simulink model "VCMGCM1962020b_v2"  (R2020b)
settings: Solver=FixedStepDiscrete  StartTime=0.0  StopTime=10.0  FixedStep=0.005  RelTol=1e-3  EnableMultiTasking=on
PreLoadFcn:
  | try, model_open; catch, disp('Error occurred while executing model pre-load callback: model_open.m'); disp('Please assure that the MATLAB working directory is set to the model directory before opening.'); end
InitFcn:
  | try, model_open; catch, end
undefined symbols (not defined in the file): Bridge, GCM, H, raptor_get_param_eval, raptor_get_safe_string, raptor_xcp_function
libraries: Blocks_lib x1165, Raptor_lib x665, simulink x62, VCM_lib x5
(part 22 of 23)

== system VCMGCM1962020b_v2/Fgnd/Actuators/CAN/Battery/ChgrBatt_State_Transition_Cmd/MsgTx/doublestrike/Falling edge ==
  In : Inport
  AND6 : Logic  AllPortsSameDT=off  OutDataTypeStr=boolean
  NOT1 : Logic  Operator=NOT  AllPortsSameDT=off  OutDataTypeStr=boolean
  Unit Delay : UnitDelay  SampleTime=-1  HasFrameUpgradeWarning=on
  falling : Outport
  wires:
  AND6/1 -> falling/1
  In/1 -> Unit Delay/1, NOT1/1
  NOT1/1 -> AND6/1
  Unit Delay/1 -> AND6/2

== system VCMGCM1962020b_v2/Fgnd/Actuators/CAN/Battery/ChgrBatt_State_Transition_Cmd/MsgTx/doublestrike/rising edge ==
  In : Inport
  AND6 : Logic  AllPortsSameDT=off  OutDataTypeStr=boolean
  NOT1 : Logic  Operator=NOT  AllPortsSameDT=off  OutDataTypeStr=boolean
  Unit Delay : UnitDelay  SampleTime=-1  HasFrameUpgradeWarning=on
  rising : Outport
  wires:
  Unit Delay/1 -> AND6/1
  NOT1/1 -> AND6/2
  AND6/1 -> rising/1
  In/1 -> NOT1/1, Unit Delay/1

== system VCMGCM1962020b_v2/Fgnd/Actuators/CAN/Battery/ChgrBatt_State_Transition_Cmd/MsgTx/doublestrike/rising edge1 ==
  In : Inport
  AND6 : Logic  AllPortsSameDT=off  OutDataTypeStr=boolean
  NOT1 : Logic  Operator=NOT  AllPortsSameDT=off  OutDataTypeStr=boolean
  Unit Delay : UnitDelay  SampleTime=-1  HasFrameUpgradeWarning=on
  rising : Outport
  wires:
  Unit Delay/1 -> AND6/1
  NOT1/1 -> AND6/2
  AND6/1 -> rising/1
  In/1 -> NOT1/1, Unit Delay/1

== system VCMGCM1962020b_v2/Fgnd/Actuators/CAN/Other/A//C Compressor/MsgName/MsgTx/Key Start ==
  Data : Inport
  Bus Selector : BusSelector  OutputSignals=Control.Other.ACC.ACCEnblReq [Bool]
  Constant : Constant  Value=uint8(0)
  Constant1 : Constant  Value=uint8(3)
  Header : Blocks_lib/Header  width=Portrait  addtext=''
  Meas&Ovrd : Blocks_lib/Meas&Ovrd  nam=[nam 'KeyStart']  name_source=Parameter  view_as=Number  enum_struct={}  gain=1  min=-inf  max=inf  precision=''  units=''  help='CAN message value'  group=['Actuators | CAN | ' msgnam]
  Multiport Switch : MultiPortSwitch  DataPortOrder=Zero-based contiguous  Inputs=2  zeroidx=on  InputSameDT=on
  enum : Outport  VectorParamsAs1DForOutWhenUnconnected=off
  wires:
  Meas&Ovrd/1 -> enum/1
  Constant/1 -> Multiport Switch/2
  Multiport Switch/1 -> Meas&Ovrd/1
  Constant1/1 -> Multiport Switch/3
  Data/1 -> Bus Selector/1
  Bus Selector/1 -> Multiport Switch/1  "<ACCEnblReq [Bool]>"

== system VCMGCM1962020b_v2/Fgnd/Actuators/CAN/Other/Power Steering Pump Inverter/PSPInvtrHC1_Demands/MsgTx/Control Word ==
  Data : Inport
  3 == Energise : Constant  Value=uint8(3)
  5 == Enable : Constant  Value=uint8(5)
  6 == Shutdown : Constant  Value=uint8(6)
  7 == Energise : simulink/Logic and Bit Operations/Compare To Constant  relop===  const=7  OutDataTypeStr=boolean
  8 == Enable : simulink/Logic and Bit Operations/Compare To Constant  relop===  const=8  OutDataTypeStr=boolean
  Bus Selector : BusSelector  OutputSignals=Control.Other.PSPInvtr.PSPInvtrEnblReq [Bool],Sensors.CAN.Other.PSPInvtr.PSPInvtrHS2_Status_Feedback.PSPInvtrInverterStatus.PSPInvtrInverterStatus [enum]
  Header : Blocks_lib/Header  width=Portrait  addtext=''
  Logical Operator : Logic  Operator=OR  OutDataTypeStr=boolean
  Meas&Ovrd : Blocks_lib/Meas&Ovrd  nam=[nam 'ControlWord']  name_source=Parameter  view_as=Number  enum_struct={}  gain=1  min=-inf  max=inf  precision=''  units='-'  help='CAN message value'  group=['Actuators | CAN | ' msgnam]
  Multiport Switch : MultiPortSwitch  DataPortOrder=Zero-based contiguous  Inputs=2  zeroidx=on  InputSameDT=on
  Multiport Switch1 : MultiPortSwitch  DataPortOrder=Zero-based contiguous  Inputs=2  zeroidx=on  InputSameDT=on
  enum : Outport  VectorParamsAs1DForOutWhenUnconnected=off
  wires:
  6 == Shutdown/1 -> Multiport Switch1/2
  Bus Selector/1 -> Multiport Switch1/1  "<PSPInvtrEnblReq [Bool]>"
  Multiport Switch/1 -> Multiport Switch1/3
  Multiport Switch1/1 -> Meas&Ovrd/1
  Logical Operator/1 -> Multiport Switch/1
  8 == Enable/1 -> Logical Operator/2
  3 == Energise/1 -> Multiport Switch/2
  5 == Enable/1 -> Multiport Switch/3
  7 == Energise/1 -> Logical Operator/1
  Bus Selector/2 -> 8 == Enable/1, 7 == Energise/1  "<PSPInvtrInverterStatus [enum]>"
  Meas&Ovrd/1 -> enum/1
  Data/1 -> Bus Selector/1

== system VCMGCM1962020b_v2/Fgnd/Control/Drive Inverter/Motor Torque Request/Driver Torque Request/Cruise Control/Control/Arbitration State ==
  PedTrq : Inport
  PIReq : Inport  Port=2
  Add : Sum
  Header : Blocks_lib/Header  width=Portrait  addtext=''
  Mux : Mux  Inputs=2
  RelOp(w/Hyst) : Blocks_lib/RelOp(w//Hyst)  relop=>=
  raptor_adjustment1 : Raptor_lib/Data Storage/raptor_adjustment  paramName='CCPedalArbHyst'  nameSource=Parameter  initValue=0  dataType=double  storage=Calibration  calDispType=Number  calEnum={}  calGain=1  calOffset=0  calMax=inf  calMin=-inf  calFormat=''  calUnit='Nm'  calHelp='Hysteresis used to determine arbitration'  calAccess=1  calFunction=group  calDispHeaders=off  calColHeaders={'Col1' 'Col2' 'Col3'}  calRowHeaders={'Row1' 'Row2' 'Row3'}
      settings: SourceProductName=Raptor
  raptor_measurement1 : Raptor_lib/Data Storage/raptor_measurement  paramName='CCPedalWinArb'  nameSource=Parameter  calDispType=Number  calEnum={'Not adapting', 'Adapting'}  calGain=1  calOffset=0  calMax=inf  calMin=-inf  calFormat=''  calUnit='Bool'  calHelp='Pedal winning arbitraion (while in cruise control)'  calAccess=1  calFunction=group  calVisible=on
      settings: SourceProductName=Raptor
  "PedWinArb " : Outport  VectorParamsAs1DForOutWhenUnconnected=off
  wires:
  RelOp(w/Hyst)/1 -> "PedWinArb "/1, raptor_measurement1/1
  PIReq/1 -> Add/2, Mux/2
  PedTrq/1 -> RelOp(w/Hyst)/1
  raptor_adjustment1/1 -> Add/1
  Add/1 -> Mux/1
  Mux/1 -> RelOp(w/Hyst)/2

== system VCMGCM1962020b_v2/Fgnd/Control/Drive Inverter/Motor Torque Request/Driver Torque Request/Cruise Control/Control/PICtrl(w//VarGain)(w//ICInport)(w//AntiWindup) ==
  Setpt : Inport
  Act : Inport  Port=2
  Rst : Inport  Port=3
  IC : Inport  Port=4
  Hold : Inport  Port=5
  Mx : Inport  Port=6
  Mn : Inport  Port=7
  Header : Blocks_lib/Header  width=Portrait  addtext=''
  PI(w/AntiWindup)(w/Hold) : Subsystem  mask(PI){samptime=samptime}
      mask prompts: samptime "Sample Time (sec)"
      mask Display: disp('PI');
  raptor_calibration1 : Raptor_lib/Data Storage/raptor_adjustment  paramName=[nam 'ErrGain']  nameSource=Parameter  initValue=0  dataType=double  storage=Calibration  calDispType=Number  calEnum={'Disabled', 'Enabled'}  calGain=1  calOffset=0  calMax=inf  calMin=-inf  calFormat=''  calUnit=[units '/' inunits]  calHelp='PID controller error gain'  calAccess=1  calFunction=group  calDispHeaders=off  calColHeaders={'Col1' 'Col2' 'Col3'}  calRowHeaders={'Row1' 'Row2' 'Row3'}
      settings: SourceProductName=Raptor
  raptor_data_def : Raptor_lib/Data Storage/raptor_data_def  dataName=[nam 'ITrm']  initValue=0  dataType=double  storage=Volatile (RAM)  calVisible=on  calType=Measurement  calDispType=Number  calEnum={'Disabled', 'Enabled'}  calGain=1  calOffset=0  calMin=-inf  calMax=inf  calFormat=''  calUnit=units  calHelp='PID controller integral term'  calAccess=1  calFunction=group  calDispHeaders=off  calColHeaders={'Col1' 'Col2' 'Col3'}  calRowHeaders={'Row1' 'Row2' 'Row3'}
      settings: SourceProductName=Raptor
  raptor_data_read : Raptor_lib/Data Storage/raptor_data_read  dataName=[nam 'ITrm']  dataShape=Scalar  idxSource=Input  idxRow=1  idxCol=1
      settings: SourceProductName=Raptor
  raptor_data_write : Raptor_lib/Data Storage/raptor_data_write  dataName=[nam 'ITrm']  dataShape=Scalar  idxSource=Write Entire Vector/Matrix  idxRow=1  idxCol=1
      settings: SourceProductName=Raptor
  raptor_interpolation_1d : Raptor_lib/Table Lookup/raptor_table_interpolate_1d  dataName=[nam 'PGainTbl']  initValue=zeros(1,dim(1))  dataType=double  storage=Calibration  adapt=off  adaptMode=Adapt between points  adaptOut=off  calVisible=on  calGain=1  calOffset=0  calMax=inf  calMin=-inf  calFormat='0.3'  calUnit='-'  calHelp='PID controller proportional gain'  calAccess=1  calFunction=group  measureEnable=on  mName=[nam 'PGain']
      settings: SourceProductName=Raptor
  raptor_interpolation_1d1 : Raptor_lib/Table Lookup/raptor_table_interpolate_1d  dataName=[nam 'IGainTbl']  initValue=zeros(1,dim(1))  dataType=double  storage=Calibration  adapt=off  adaptMode=Adapt between points  adaptOut=off  calVisible=on  calGain=1  calOffset=0  calMax=inf  calMin=-inf  calFormat='0.3'  calUnit='1/sec'  calHelp='PID controller integral gain'  calAccess=1  calFunction=group  measureEnable=on  mName=[nam 'IGain']
      settings: SourceProductName=Raptor
  raptor_prelookup4 : Raptor_lib/Table Lookup/raptor_table_axis  dataName=[nam 'Err' num2str(dim(1)) 'IdxArr']  initValue=[1:dim(1)]  dataType=double  storage=Calibration  calVisible=on  calGain=1  calOffset=0  calMax=inf  calMin=-inf  calFormat=''  calUnit=inunits  calHelp='Index array'  calAccess=1  calFunction=group
      settings: SourceProductName=Raptor
  raptor_probe : Raptor_lib/Data Storage/raptor_measurement  paramName=[nam 'ErrTrm']  nameSource=Parameter  calDispType=Number  calEnum={'Disabled', 'Enabled'}  calGain=1  calOffset=0  calMax=inf  calMin=-inf  calFormat=''  calUnit=inunits  calHelp='PID controller error term'  calAccess=1  calFunction=group  calVisible=on
      settings: SourceProductName=Raptor
  raptor_probe1 : Raptor_lib/Data Storage/raptor_measurement  paramName=[nam 'PTrm']  nameSource=Parameter  calDispType=Number  calEnum={'Disabled', 'Enabled'}  calGain=1  calOffset=0  calMax=inf  calMin=-inf  calFormat=''  calUnit=units  calHelp='PID controller proportional term'  calAccess=1  calFunction=group  calVisible=on
      settings: SourceProductName=Raptor
  raptor_probe6 : Raptor_lib/Data Storage/raptor_measurement  paramName=[nam 'Cmd']  nameSource=Parameter  calDispType=Number  calEnum={'Disabled', 'Enabled'}  calGain=1  calOffset=0  calMax=inf  calMin=-inf  calFormat=''  calUnit=units  calHelp='PID controller output'  calAccess=1  calFunction=group  calVisible=on
      settings: SourceProductName=Raptor
  Cmd : Outport  VectorParamsAs1DForOutWhenUnconnected=off
  wires:
  Rst/1 -> PI(w/AntiWindup)(w/Hold)/6(Rst)
  Act/1 -> PI(w/AntiWindup)(w/Hold)/2(Act)
  Setpt/1 -> PI(w/AntiWindup)(w/Hold)/1(Setpt)
  raptor_calibration1/1 -> PI(w/AntiWindup)(w/Hold)/3(kErr)
  IC/1 -> PI(w/AntiWindup)(w/Hold)/7(IC)
  PI(w/AntiWindup)(w/Hold)/3(PTerm) -> raptor_probe1/1
  PI(w/AntiWindup)(w/Hold)/1(Out) -> Cmd/1, raptor_probe6/1
  raptor_interpolation_1d/1 -> PI(w/AntiWindup)(w/Hold)/4(kP)
  raptor_interpolation_1d1/1 -> PI(w/AntiWindup)(w/Hold)/5(kI)
  raptor_prelookup4/1 -> raptor_interpolation_1d/1, raptor_interpolation_1d1/1
  raptor_data_read/1 -> PI(w/AntiWindup)(w/Hold)/11(PrevITrm)
  PI(w/AntiWindup)(w/Hold)/4(ITrm) -> raptor_data_write/1
  PI(w/AntiWindup)(w/Hold)/2(Err) -> raptor_prelookup4/1, raptor_probe/1
  Mx/1 -> PI(w/AntiWindup)(w/Hold)/9(Mx)
  Mn/1 -> PI(w/AntiWindup)(w/Hold)/10(Mn)
  Hold/1 -> PI(w/AntiWindup)(w/Hold)/8(Hold)

== system VCMGCM1962020b_v2/Fgnd/Control/Drive Inverter/Motor Torque Request/Driver Torque Request/Cruise Control/Control/Reset, IC, & Limits ==
  note: Note: This is the previous time-step
      | final torque request.
  note: Note:
      | On the first time step (ie, cruise control becoming active), the integral term is pre-loaded at (LastTrqReq - FFTerm).
      | Then, when the feedforward term and PTerm is added, the initial output of the complete controller is (LastTrqReq + PTerm).
      |
      | When the pedal is winning arbitration , the idle PI controller’s integral term is also reset to (LastTrqReq – FFTerm).
      | Then, when the feedforward term and PTerm is added, the output of the complete controller is (LastTrqReq + PTerm).
  Data : Inport
  Setpt : Inport  Port=2
  FF : Inport  Port=3
  PedWinArb : Inport  Port=4
  Add1 : Sum  Inputs=+-
  Add2 : Sum  Inputs=+-
  Add3 : Sum  Inputs=+-
  Bus Selector : BusSelector  OutputSignals=Control.DrvInvtr.MtrTrqReq.DrvInvtr.DrvMtrTrqLim [Nm]
  Bus Selector1 : BusSelector  OutputSignals=Control.DrvInvtr.MtrTrqReq.DrvInvtr.DrvMtrTrqReq [Nm]
  Demux : Demux  Outputs=2
  FirstTS : Blocks_lib/FirstTS  SystemSampleTime=-1  VariantActivationTime=update diagram  Latency=0  AutoFrameSizeCalculation=off
  Header : Blocks_lib/Header  width=Portrait  addtext=''
  Logical Operator : Logic  Operator=OR  AllPortsSameDT=off  OutDataTypeStr=boolean
  Speed Pulled High : Subsystem
  Unit Delay : UnitDelay  SampleTime=-1  HasFrameUpgradeWarning=on
  Rst : Outport  VectorParamsAs1DForOutWhenUnconnected=off
  " IC " : Outport  Port=2  VectorParamsAs1DForOutWhenUnconnected=off
  " Hold" : Outport  Port=3  VectorParamsAs1DForOutWhenUnconnected=off
  Mx : Outport  Port=4  VectorParamsAs1DForOutWhenUnconnected=off
  Mn : Outport  Port=5  VectorParamsAs1DForOutWhenUnconnected=off
  wires:
  Unit Delay/1 -> Add1/1
  Add3/1 -> Mn/1
  Bus Selector1/1 -> Unit Delay/1  "<DrvMtrTrqReq [Nm]>"
  Add2/1 -> Mx/1
  Add1/1 -> " IC "/1
  Demux/1 -> Add2/1
  FirstTS/1 -> Logical Operator/1
  FF/1 -> Add1/2, Add3/2, Add2/2
  PedWinArb/1 -> Logical Operator/2, Speed Pulled High/3(PedWinArb)
  Logical Operator/1 -> Rst/1
  Speed Pulled High/1(Bool) -> " Hold"/1
  Setpt/1 -> Speed Pulled High/2(Setpt)
  Demux/2 -> Add3/1
  Bus Selector/1 -> Demux/1  "<DrvMtrTrqLim [Nm]>"
  Data/1 -> Bus Selector1/1, Speed Pulled High/1(Data), Bus Selector/1

== system VCMGCM1962020b_v2/Fgnd/Control/Drive Inverter/Motor Torque Request/Driver Torque Request/Cruise Control/Setpoint/Enable ==
  Data : Inport
  Bus Selector : BusSelector  OutputSignals=Control.Mode.PRNDMode [enum]
  Bus Selector1 : BusSelector  OutputSignals=VirtualSensors.Spd.VehDir [enum]
  Bus Selector2 : BusSelector  OutputSignals=VirtualSensors.Spd.VehSpd [kph]
  CmprTo : Blocks_lib/CmprTo  op===  val='Drv'  enum=EnumLst.PRNDMode
  CmprTo1 : Blocks_lib/CmprTo  op===  val='Fwd'  enum=EnumLst.VehDir
  Header : Blocks_lib/Header  width=Portrait  addtext=''
  Logical Operator : Logic  Inputs=1  OutDataTypeStr=boolean
  Logical Operator1 : Logic  Operator=NOT  Inputs=1  OutDataTypeStr=boolean
  Mux : Mux  Inputs=5
  Relational Operator : RelationalOperator  Operator=<=  OutDataTypeStr=boolean  RndMeth=Simplest
  raptor_adjustment : Raptor_lib/Data Storage/raptor_adjustment  paramName='CCEnbl_cal'  nameSource=Parameter  initValue=0  dataType=boolean  storage=Calibration  calDispType=Number  calEnum={'False', 'True'}  calGain=1  calOffset=0  calMax=inf  calMin=-inf  calFormat=''  calUnit='Bool'  calHelp='Cruise control enable'  calAccess=1  calFunction=group  calDispHeaders=off  calColHeaders={'Col1' 'Col2' 'Col3'}  calRowHeaders={'Row1' 'Row2' 'Row3'}
      settings: SourceProductName=Raptor
  raptor_adjustment1 : Raptor_lib/Data Storage/raptor_adjustment  paramName='CCVehSpdHiThr'  nameSource=Parameter  initValue=0  dataType=double  storage=Calibration  calDispType=Number  calEnum={'False', 'True'}  calGain=1  calOffset=0  calMax=inf  calMin=-inf  calFormat=''  calUnit='kph'  calHelp='Cruise control enable vehicle speed high threshold'  calAccess=1  calFunction=group  calDispHeaders=off  calColHeaders={'Col1' 'Col2' 'Col3'}  calRowHeaders={'Row1' 'Row2' 'Row3'}
      settings: SourceProductName=Raptor
  raptor_fault_action : Raptor_lib/Faults/raptor_fault_action  actionName='CCDsbl'  calVisible=off  calAccess=1  calFunction='System | FaultManager | FaultAction'
      settings: SourceProductName=Raptor
  raptor_measurement : Raptor_lib/Data Storage/raptor_measurement  paramName='CCEnbl'  nameSource=Parameter  calDispType=Number  calEnum={}  calGain=1  calOffset=0  calMax=inf  calMin=-inf  calFormat=''  calUnit='Bool'  calHelp='Cruise control enable criteria met'  calAccess=1  calFunction=group  calVisible=on
      settings: SourceProductName=Raptor
  Enbl : Outport  VectorParamsAs1DForOutWhenUnconnected=off
  wires:
  CmprTo/1 -> Mux/3
  Bus Selector/1 -> CmprTo/1  "<PRNDMode [enum]>"
  Mux/1 -> raptor_measurement/1, Logical Operator/1
  Relational Operator/1 -> Mux/5
  raptor_adjustment1/1 -> Relational Operator/2
  raptor_adjustment/1 -> Mux/1
  Bus Selector2/1 -> Relational Operator/1  "<VehSpd [kph]>"
  Logical Operator1/1 -> Mux/2
  Logical Operator/1 -> Enbl/1
  raptor_fault_action/1 -> Logical Operator1/1
  Data/1 -> Bus Selector/1, Bus Selector1/1, Bus Selector2/1
  Bus Selector1/1 -> CmprTo1/1  "<VehDir [enum]>"
  CmprTo1/1 -> Mux/4

== system VCMGCM1962020b_v2/Fgnd/Control/Drive Inverter/Motor Torque Request/Driver Torque Request/Cruise Control/Setpoint/SetptMnMx ==
  Data : Inport
  Add : Sum  Inputs=+-
  Add1 : Sum
  Bus Selector : BusSelector  OutputSignals=Control.DrvInvtr.MtrTrqReq.DrvTrqReq.VehSpdLim [kph]
  Header : Blocks_lib/Header  width=Portrait  addtext=''
  MinMax : MinMax  Inputs=2
  raptor_adjustment : Raptor_lib/Data Storage/raptor_adjustment  paramName='CCSetptMnMxDelta'  nameSource=Parameter  initValue=0  dataType=double  storage=Calibration  calDispType=Number  calEnum={'False', 'True'}  calGain=1  calOffset=0  calMax=inf  calMin=-inf  calFormat=''  calUnit='kph'  calHelp='Cruise control setpoint minimum/maximum delta (relative to high/low thresholds)'  calAccess=1  calFunction=group  calDispHeaders=off  calColHeaders={'Col1' 'Col2' 'Col3'}  calRowHeaders={'Row1' 'Row2' 'Row3'}
      settings: SourceProductName=Raptor
  raptor_data_read : Raptor_lib/Data Storage/raptor_data_read  dataName='CCVehSpdLoThr'  dataShape=Scalar  idxSource=Read Entire Vector/Matrix  idxRow=1  idxCol=1
      settings: SourceProductName=Raptor
  raptor_data_read1 : Raptor_lib/Data Storage/raptor_data_read  dataName='CCVehSpdHiThr'  dataShape=Scalar  idxSource=Read Entire Vector/Matrix  idxRow=1  idxCol=1
      settings: SourceProductName=Raptor
  Mx : Outport  VectorParamsAs1DForOutWhenUnconnected=off
  Mn : Outport  Port=2  VectorParamsAs1DForOutWhenUnconnected=off
  wires:
  raptor_adjustment/1 -> Add/2, Add1/1
  Add/1 -> MinMax/2
  Bus Selector/1 -> MinMax/1  "<VehSpdLim [kph]>"
  Data/1 -> Bus Selector/1
  Add1/1 -> Mn/1
  MinMax/1 -> Mx/1
  raptor_data_read/1 -> Add1/2
  raptor_data_read1/1 -> Add/1

== system VCMGCM1962020b_v2/Fgnd/Control/Drive Inverter/Motor Torque Request/Driver Torque Request/Cruise Control/Setpoint/Standby ==
  Data : Inport
  Bus Selector : BusSelector  OutputSignals=VirtualSensors.Driver.BrkSw [Bool]
  Bus Selector1 : BusSelector  OutputSignals=VirtualSensors.Driver.CCCancel [Bool]
  Bus Selector2 : BusSelector  OutputSignals=VirtualSensors.Spd.VehSpd [kph]
  Header : Blocks_lib/Header  width=Portrait  addtext=''
  Logical Operator : Logic  Operator=OR  Inputs=1  OutDataTypeStr=boolean
  Mux : Mux  Inputs=3
  Relational Operator : RelationalOperator  Operator=<  OutDataTypeStr=boolean  RndMeth=Simplest
  raptor_adjustment : Raptor_lib/Data Storage/raptor_adjustment  paramName='CCVehSpdLoThr'  nameSource=Parameter  initValue=0  dataType=double  storage=Calibration  calDispType=Number  calEnum={'False', 'True'}  calGain=1  calOffset=0  calMax=inf  calMin=-inf  calFormat=''  calUnit='kph'  calHelp='Cruise control enable vehicle speed low threshold'  calAccess=1  calFunction=group  calDispHeaders=off  calColHeaders={'Col1' 'Col2' 'Col3'}  calRowHeaders={'Row1' 'Row2' 'Row3'}
      settings: SourceProductName=Raptor
  raptor_measurement : Raptor_lib/Data Storage/raptor_measurement  paramName='CCStndby'  nameSource=Parameter  calDispType=Number  calEnum={}  calGain=1  calOffset=0  calMax=inf  calMin=-inf  calFormat=''  calUnit='Bool'  calHelp='Cruise control in standby'  calAccess=1  calFunction=group  calVisible=on
      settings: SourceProductName=Raptor
  Stndby : Outport  VectorParamsAs1DForOutWhenUnconnected=off
  wires:
  Bus Selector1/1 -> Mux/2  "<CCCancel [Bool]>"
  Logical Operator/1 -> Stndby/1
  raptor_adjustment/1 -> Relational Operator/2
  Bus Selector2/1 -> Relational Operator/1  "<VehSpd [kph]>"
  Bus Selector/1 -> Mux/1  "<BrkSw [Bool]>"
  Relational Operator/1 -> Mux/3
  Mux/1 -> raptor_measurement/1, Logical Operator/1
  Data/1 -> Bus Selector/1, Bus Selector1/1, Bus Selector2/1

== system VCMGCM1962020b_v2/Fgnd/Control/Drive Inverter/Motor Torque Request/Inverter//Motor Limit & Request/Motor Torque Request/Gearbox Preload/Preload Initialize ==
  Data : Inport
  TrqReq : Inport  Port=2
  Bus Selector : BusSelector  OutputSignals=Control.Mode.PRNDMode [enum]
  CmprTo : Blocks_lib/CmprTo  op===  val='Rev'  enum=EnumLst.PRNDMode
  CmprTo1 : Blocks_lib/CmprTo  op===  val='Drv'  enum=EnumLst.PRNDMode
  Combinatorial Logic : CombinatorialLogic  TruthTable=[0; 2; 1; 0]
  Compare To Zero : simulink/Logic and Bit Operations/Compare To Zero  relop=<=  OutDataTypeStr=boolean
  Compare To Zero1 : simulink/Logic and Bit Operations/Compare To Zero  relop=>=  OutDataTypeStr=boolean
  Detect Increase{,1..3} (4 alike) : simulink/Logic and Bit Operations/Detect Increase  vinit=0.0  OutDataTypeStr=boolean
  Header : Blocks_lib/Header  width=Portrait  addtext=''
  Logical Operator : Logic  Operator=OR  AllPortsSameDT=off  OutDataTypeStr=boolean
  Logical Operator1 : Logic  AllPortsSameDT=off  OutDataTypeStr=boolean
  Logical Operator2 : Logic  Operator=OR  AllPortsSameDT=off  OutDataTypeStr=boolean
  Logical Operator3 : Logic  AllPortsSameDT=off  OutDataTypeStr=boolean
  Mux : Mux  Inputs=2
  enum : Outport  VectorParamsAs1DForOutWhenUnconnected=off
  wires:
  CmprTo1/1 -> Logical Operator3/1, Detect Increase1/1
  CmprTo/1 -> Logical Operator1/1, Detect Increase/1
  Logical Operator/1 -> Mux/1
  Logical Operator2/1 -> Mux/2
  Logical Operator3/1 -> Logical Operator2/2
  Compare To Zero1/1 -> Detect Increase3/1
  Detect Increase3/1 -> Logical Operator3/2
  Detect Increase2/1 -> Logical Operator1/2
  Compare To Zero/1 -> Detect Increase2/1
  TrqReq/1 -> Compare To Zero/1, Compare To Zero1/1
  Logical Operator1/1 -> Logical Operator/2
  Combinatorial Logic/1 -> enum/1
  Mux/1 -> Combinatorial Logic/1
  Detect Increase1/1 -> Logical Operator2/1
  Detect Increase/1 -> Logical Operator/1
  Data/1 -> Bus Selector/1
  Bus Selector/1 -> CmprTo1/1, CmprTo/1  "<PRNDMode [enum]>"

== system VCMGCM1962020b_v2/Fgnd/Control/Drive Inverter/Motor Torque Request/Inverter//Motor Limit & Request/Motor Torque Request/Rate Limit/RateLim ==
  Prev : Inport
  Rst : Inport  Port=2
  In : Inport  Port=3
  "[+R -R]" : Inport  Port=4
  Add : Sum  Inputs=+-  InputSameDT=on  OutDataTypeStr=Inherit: Same as first input
  Add1 : Sum  InputSameDT=on  OutDataTypeStr=Inherit: Same as first input
  Constant : Constant  Value=double(samptime)
  Constant1 : Constant  Value=double(0)
  Header : Blocks_lib/Header  width=Portrait  addtext=''
  Multiport Switch : MultiPortSwitch  DataPortOrder=Zero-based contiguous  Inputs=2  zeroidx=on  InputSameDT=on
  Product : Product  OutDataTypeStr=Inherit: Inherit via back propagation  RndMeth=Zero
  Sat : Subsystem  mask(Sat){}
      mask Display: plot([0.4 0.5 0.6 0.7], [0.1 0.1 0.9 0.9]);
  Out : Outport  VectorParamsAs1DForOutWhenUnconnected=off
  wires:
  Constant1/1 -> Multiport Switch/3
  In/1 -> Add/1
  Product/1 -> Sat/2("[Mx Mn]")
  Constant/1 -> Product/2
  "[+R -R]"/1 -> Product/1
  Rst/1 -> Multiport Switch/1
  Add1/1 -> Multiport Switch/2
  Multiport Switch/1 -> Out/1
  Sat/1(Out) -> Add1/2
  Add/1 -> Sat/1(In)
  Prev/1 -> Add1/1, Add/2

== system VCMGCM1962020b_v2/Fgnd/Virtual Sensors/PDU/HVBusVolt/HV Bus Voltage/Sum, Max, Min/Loop/Data Valid ==
  V : Inport
  Enable : EnablePort
  Add : Sum
  Add1 : Sum
  Constant : Constant  Value=uint8(1)
  Header : Blocks_lib/Header  width=Portrait  addtext=''
  MinMax : MinMax  Function=max  Inputs=2
  MinMax1 : MinMax  Inputs=2
  raptor_data_def : Raptor_lib/Data Storage/raptor_data_def  dataName=[nam 'Sum']  initValue=0  dataType=double  storage=Volatile (RAM)  calVisible=off  calType=Measurement  calDispType=Number  calEnum={'False', 'True'}  calGain=1.0  calOffset=0  calMin=-inf  calMax=inf  calFormat='-1'  calUnit=''  calHelp=''  calAccess=1  calFunction=raptor_xcp_function(gcb)  calDispHeaders=off  calColHeaders={'Col1' 'Col2' 'Col3'}  calRowHeaders={'Row1' 'Row2' 'Row3'}
      settings: SourceProductName=Raptor
  raptor_data_def1 : Raptor_lib/Data Storage/raptor_data_def  dataName=[nam 'Mx']  initValue=0  dataType=double  storage=Volatile (RAM)  calVisible=off  calType=Measurement  calDispType=Number  calEnum={'False', 'True'}  calGain=1.0  calOffset=0  calMin=-inf  calMax=inf  calFormat='-1'  calUnit=''  calHelp=''  calAccess=1  calFunction=raptor_xcp_function(gcb)  calDispHeaders=off  calColHeaders={'Col1' 'Col2' 'Col3'}  calRowHeaders={'Row1' 'Row2' 'Row3'}
      settings: SourceProductName=Raptor
  raptor_data_def2 : Raptor_lib/Data Storage/raptor_data_def  dataName=[nam 'Mn']  initValue=0  dataType=double  storage=Volatile (RAM)  calVisible=off  calType=Measurement  calDispType=Number  calEnum={'False', 'True'}  calGain=1.0  calOffset=0  calMin=-inf  calMax=inf  calFormat='-1'  calUnit=''  calHelp=''  calAccess=1  calFunction=raptor_xcp_function(gcb)  calDispHeaders=off  calColHeaders={'Col1' 'Col2' 'Col3'}  calRowHeaders={'Row1' 'Row2' 'Row3'}
      settings: SourceProductName=Raptor
  raptor_data_def3 : Raptor_lib/Data Storage/raptor_data_def  dataName=[nam 'SumCount']  initValue=0  dataType=uint8  storage=Volatile (RAM)  calVisible=off  calType=Measurement  calDispType=Number  calEnum={'False', 'True'}  calGain=1.0  calOffset=0  calMin=-inf  calMax=inf  calFormat='-1'  calUnit=''  calHelp=''  calAccess=1  calFunction=raptor_xcp_function(gcb)  calDispHeaders=off  calColHeaders={'Col1' 'Col2' 'Col3'}  calRowHeaders={'Row1' 'Row2' 'Row3'}
      settings: SourceProductName=Raptor
  raptor_data_read : Raptor_lib/Data Storage/raptor_data_read  dataName=[nam 'Sum']  dataShape=Scalar  idxSource=Input  idxRow=1  idxCol=1
      settings: SourceProductName=Raptor
  raptor_data_read1 : Raptor_lib/Data Storage/raptor_data_read  dataName=[nam 'Mx']  dataShape=Scalar  idxSource=Input  idxRow=1  idxCol=1
      settings: SourceProductName=Raptor
  raptor_data_read2 : Raptor_lib/Data Storage/raptor_data_read  dataName=[nam 'Mn']  dataShape=Scalar  idxSource=Input  idxRow=1  idxCol=1
      settings: SourceProductName=Raptor
  raptor_data_read3 : Raptor_lib/Data Storage/raptor_data_read  dataName=[nam 'SumCount']  dataShape=Scalar  idxSource=Input  idxRow=1  idxCol=1
      settings: SourceProductName=Raptor
  raptor_data_write : Raptor_lib/Data Storage/raptor_data_write  dataName=[nam 'Sum']  dataShape=Scalar  idxSource=Input Port  idxRow=1  idxCol=1
      settings: SourceProductName=Raptor
  raptor_data_write1 : Raptor_lib/Data Storage/raptor_data_write  dataName=[nam 'Mx']  dataShape=Scalar  idxSource=Input Port  idxRow=1  idxCol=1
      settings: SourceProductName=Raptor
  raptor_data_write2 : Raptor_lib/Data Storage/raptor_data_write  dataName=[nam 'Mn']  dataShape=Scalar  idxSource=Input Port  idxRow=1  idxCol=1
      settings: SourceProductName=Raptor
  raptor_data_write3 : Raptor_lib/Data Storage/raptor_data_write  dataName=[nam 'SumCount']  dataShape=Scalar  idxSource=Input Port  idxRow=1  idxCol=1
      settings: SourceProductName=Raptor
  wires:
  raptor_data_read/1 -> Add/1
  Add/1 -> raptor_data_write/1
  raptor_data_read1/1 -> MinMax/1
  MinMax/1 -> raptor_data_write1/1
  MinMax1/1 -> raptor_data_write2/1
  raptor_data_read2/1 -> MinMax1/1
  V/1 -> Add/2, MinMax/2, MinMax1/2
  Add1/1 -> raptor_data_write3/1
  raptor_data_read3/1 -> Add1/1
  Constant/1 -> Add1/2

== system VCMGCM1962020b_v2/Fgnd/Control/Drive Inverter/Motor Torque Request/Driver Torque Request/Cruise Control/Control/PICtrl(w//VarGain)(w//ICInport)(w//AntiWindup)/PI(w//AntiWindup)(w//Hold) ==
  Setpt : Inport
  Act : Inport  Port=2
  kErr : Inport  Port=3
  kP : Inport  Port=4
  kI : Inport  Port=5
  Rst : Inport  Port=6
  IC : Inport  Port=7
  Hold : Inport  Port=8
  Mx : Inport  Port=9
  Mn : Inport  Port=10
  PrevITrm : Inport  Port=11
  Add : Sum  Inputs=+-  InputSameDT=on  OutDataTypeStr=Inherit: Same as first input
  Add1 : Sum  Inputs=+-  InputSameDT=on  OutDataTypeStr=Inherit: Same as first input
  Add2 : Sum  Inputs=+-  InputSameDT=on  OutDataTypeStr=Inherit: Same as first input
  Header : Blocks_lib/Header  width=Portrait  addtext=''
  Intgl(w/Hold) : Subsystem  mask(Intgl){samptime=samptime}
      mask prompts: samptime "Sample Time (sec)"
      mask Display: disp('Integral');
  Multiport Switch : MultiPortSwitch  DataPortOrder=Zero-based contiguous  Inputs=2  zeroidx=on
  Multiport Switch1 : MultiPortSwitch  DataPortOrder=Zero-based contiguous  Inputs=2  zeroidx=on
  Mux : Mux  Inputs=2
  Product1 : Product  InputSameDT=on  OutDataTypeStr=Inherit: Same as first input
  Product2 : Product  InputSameDT=on  OutDataTypeStr=Inherit: Same as first input
  Product5 : Product  InputSameDT=on  OutDataTypeStr=Inherit: Same as first input
  Sat : Blocks_lib/Sat  SystemSampleTime=-1  VariantActivationTime=update diagram  Latency=0  AutoFrameSizeCalculation=off
  Sum1 : Sum  Inputs=+|+  InputSameDT=on  SaturateOnIntegerOverflow=on  OutDataTypeStr=Inherit: Same as first input
  Out : Outport  VectorParamsAs1DForOutWhenUnconnected=off
  Err : Outport  Port=2  VectorParamsAs1DForOutWhenUnconnected=off
  PTerm : Outport  Port=3  VectorParamsAs1DForOutWhenUnconnected=off
  ITrm : Outport  Port=4  VectorParamsAs1DForOutWhenUnconnected=off
  wires:
  Multiport Switch1/1 -> Intgl(w/Hold)/6(Mn)
  Multiport Switch/1 -> Intgl(w/Hold)/5(Mx)
  Rst/1 -> Multiport Switch1/1, Multiport Switch/1, Intgl(w/Hold)/2(Rst)
  IC/1 -> Intgl(w/Hold)/3(IC)
  Product1/1 -> Intgl(w/Hold)/1(In)
  Mx/1 -> Mux/1, Multiport Switch/3, Add1/1
  Mn/1 -> Mux/2, Add2/1, Multiport Switch1/3
  PrevITrm/1 -> Intgl(w/Hold)/7(PrevOut)
  Add/1 -> Product5/1, Err/1
  kErr/1 -> Product5/2
  Act/1 -> Add/2
  kP/1 -> Product2/2
  kI/1 -> Product1/2
  Sum1/1 -> Out/1
  Product5/1 -> Product2/1, Product1/1
  Setpt/1 -> Add/1
  Intgl(w/Hold)/1(Out) -> Sum1/2, ITrm/1
  Product2/1 -> Sat/1
  Add1/1 -> Multiport Switch/2
  Add2/1 -> Multiport Switch1/2
  Mux/1 -> Sat/2
  Sat/1 -> Add2/2, Add1/2, Sum1/1, PTerm/1
  Hold/1 -> Intgl(w/Hold)/4(Hold)

== system VCMGCM1962020b_v2/Fgnd/Control/Drive Inverter/Motor Torque Request/Driver Torque Request/Cruise Control/Control/Reset, IC, & Limits/Speed Pulled High ==
  Data : Inport
  Setpt : Inport  Port=2
  PedWinArb : Inport  Port=3
  Add : Sum  Inputs=+-
  Bus Selector1 : BusSelector  OutputSignals=VirtualSensors.Spd.VehSpd [kph]
  Bus Selector2 : BusSelector  OutputSignals=CCSetpt [kph]
  Header : Blocks_lib/Header  width=Portrait  addtext=''
  Logical Operator1 : Logic  Operator=NOT  Inputs=1  AllPortsSameDT=off  OutDataTypeStr=boolean
  Logical Operator3 : Logic  AllPortsSameDT=off  OutDataTypeStr=boolean
  Logical Operator7 : Logic  Operator=NOT  Inputs=1  AllPortsSameDT=off  OutDataTypeStr=boolean
  Relational Operator : RelationalOperator  Operator=<=  OutDataTypeStr=boolean  RndMeth=Nearest
  raptor_adjustment1 : Raptor_lib/Data Storage/raptor_adjustment  paramName='CCSpdInRangeThr'  nameSource=Parameter  initValue=0  dataType=double  storage=Calibration  calDispType=Number  calEnum={'False', 'True'}  calGain=1  calOffset=0  calMax=inf  calMin=-inf  calFormat=''  calUnit='kph'  calHelp='Cruise control speed in range threshold'  calAccess=1  calFunction=group  calDispHeaders=off  calColHeaders={'Col1' 'Col2' 'Col3'}  calRowHeaders={'Row1' 'Row2' 'Row3'}
      settings: SourceProductName=Raptor
  raptor_measurement1 : Raptor_lib/Data Storage/raptor_measurement  paramName='CCSpdInRange'  nameSource=Parameter  calDispType=Number  calEnum={'Not adapting', 'Adapting'}  calGain=1  calOffset=0  calMax=inf  calMin=-inf  calFormat=''  calUnit='Bool'  calHelp='Cruise control speed in range'  calAccess=1  calFunction=group  calVisible=on
      settings: SourceProductName=Raptor
  raptor_measurement3 : Raptor_lib/Data Storage/raptor_measurement  paramName='CCSpdPulledHigh'  nameSource=Parameter  calDispType=Number  calEnum={'Not adapting', 'Adapting'}  calGain=1  calOffset=0  calMax=inf  calMin=-inf  calFormat=''  calUnit='Bool'  calHelp='Cruise control speed pulled high (eg, due to coasting)'  calAccess=1  calFunction=group  calVisible=on
      settings: SourceProductName=Raptor
  Bool : Outport  VectorParamsAs1DForOutWhenUnconnected=off
  wires:
  Logical Operator3/1 -> raptor_measurement3/1, Bool/1
  Logical Operator7/1 -> Logical Operator3/1
  PedWinArb/1 -> Logical Operator1/1
  Logical Operator1/1 -> Logical Operator3/2
  Add/1 -> Relational Operator/1
  Bus Selector1/1 -> Add/1  "<VehSpd [kph]>"
  raptor_adjustment1/1 -> Relational Operator/2
  Bus Selector2/1 -> Add/2  "<CCSetpt [kph]>"
  Setpt/1 -> Bus Selector2/1
  Data/1 -> Bus Selector1/1
  Relational Operator/1 -> raptor_measurement1/1, Logical Operator7/1

== system VCMGCM1962020b_v2/Fgnd/Control/Drive Inverter/Motor Torque Request/Inverter//Motor Limit & Request/Motor Torque Request/Rate Limit/RateLim/Sat ==
  In : Inport
  "[Mx Mn]" : Inport  Port=2
  Header : Blocks_lib/Header  width=Portrait  addtext=''
  MinMax : MinMax  Function=max  InputSameDT=on  SaturateOnIntegerOverflow=on  ZeroCross=off
  MinMax1 : MinMax  InputSameDT=on  SaturateOnIntegerOverflow=on  ZeroCross=off
  MinMax2 : MinMax  Inputs=2  InputSameDT=on  SaturateOnIntegerOverflow=on  ZeroCross=off
  MinMax3 : MinMax  Function=max  Inputs=2  InputSameDT=on  SaturateOnIntegerOverflow=on  ZeroCross=off
  Saturation : Saturate  UpperLimit=inf  LowerLimit=0
  Saturation1 : Saturate  UpperLimit=0  LowerLimit=-inf
  Out : Outport  VectorParamsAs1DForOutWhenUnconnected=off
  wires:
  Saturation1/1 -> MinMax3/2
  Saturation/1 -> MinMax2/2
  MinMax3/1 -> Out/1
  In/1 -> MinMax2/1
  MinMax2/1 -> MinMax3/1
  MinMax/1 -> Saturation/1
  MinMax1/1 -> Saturation1/1
  "[Mx Mn]"/1 -> MinMax/1, MinMax1/1

== system VCMGCM1962020b_v2/Fgnd/Control/Drive Inverter/Motor Torque Request/Driver Torque Request/Cruise Control/Control/PICtrl(w//VarGain)(w//ICInport)(w//AntiWindup)/PI(w//AntiWindup)(w//Hold)/Intgl(w//Hold) ==
  In : Inport
  Rst : Inport  Port=2
  IC : Inport  Port=3
  Hold : Inport  Port=4
  Mx : Inport  Port=5
  Mn : Inport  Port=6
  PrevOut : Inport  Port=7
  Add1 : Sum  InputSameDT=on  OutDataTypeStr=Inherit: Same as first input
  Constant : Constant  Value=double(samptime)
  Header : Blocks_lib/Header  width=Portrait  addtext=''
  Multiport Switch1 : MultiPortSwitch  DataPortOrder=Zero-based contiguous  Inputs=2  zeroidx=on  InputSameDT=on
  Multiport Switch3 : MultiPortSwitch  DataPortOrder=Zero-based contiguous  Inputs=2  zeroidx=on  InputSameDT=on
  Mux : Mux  Inputs=2
  Product1 : Product  SaturateOnIntegerOverflow=on  OutDataTypeStr=Inherit: Same as first input
  Sat : Blocks_lib/Sat  SystemSampleTime=-1  VariantActivationTime=update diagram  Latency=0  AutoFrameSizeCalculation=off
  Out : Outport  VectorParamsAs1DForOutWhenUnconnected=off
  wires:
  Mux/1 -> Sat/2
  Mn/1 -> Mux/2
  Mx/1 -> Mux/1
  PrevOut/1 -> Multiport Switch1/3, Add1/1
  Add1/1 -> Multiport Switch1/2
  Sat/1 -> Out/1
  Multiport Switch3/1 -> Sat/1
  In/1 -> Product1/1
  Product1/1 -> Add1/2
  IC/1 -> Multiport Switch3/3
  Rst/1 -> Multiport Switch3/1
  Constant/1 -> Product1/2
  Hold/1 -> Multiport Switch1/1
  Multiport Switch1/1 -> Multiport Switch3/2

== stateflow chart VCMGCM1962020b_v2/Fgnd/Control/Other/Other/FMWS/Chart1 ==
  (junction 11) -> (junction 13) : {FMWS_State_gear = 130 }
  (junction 3) -> (junction 11) [order 1] : [Drv == 1]
  (junction 15) -> (junction 17) : {FMWS_State_gear = 125 }
  (junction 3) -> (junction 15) [order 2] : [Ntrl == 1]
  (default) -> (junction 3)
  (junction 3) -> (junction 21) [order 3] : [Rev ==1]
  (junction 3) -> (junction 55) [order 4] : [Prk == 1]
  (junction 21) -> (junction 19) : {FMWS_State_gear = 120}
  (junction 55) -> (junction 54) : {FMWS_State_gear = 251}
  data: Drv input; Ntrl input; Rev input; FMWS_State_gear output; Prk input

== stateflow chart VCMGCM1962020b_v2/Fgnd/Control/Modes/PRND Mode/PRND_FMWS ==
  (junction 5) -> (junction 17) : {PRND_Act_Out = 251}
  (junction 3) -> (junction 5) [order 1] : [PRND_In == 0]
  (junction 6) -> (junction 13) : {PRND_Act_Out = -125}
  (junction 3) -> (junction 6) [order 2] : [PRND_In == 1]
  (default) -> (junction 3)
  (junction 3) -> (junction 7) [order 3] : [PRND_In == 3]
  (junction 3) -> (junction 8) [order 4] : [PRND_In == 2]
  (junction 7) -> (junction 15) : {PRND_Act_Out = 126}
  (junction 8) -> (junction 19) : {PRND_Act_Out = 125}
  data: PRND_In input; PRND_Act_Out output

== stateflow chart VCMGCM1962020b_v2/Fgnd/Control/Modes/PRND Mode/PRND Mode ==
  state PARK
    en: PRNDMode = 0
  state NOT_PARK
    state REVERSE
      en: PRNDMode = 1
    state NEUTRAL
      en: PRNDMode = 2
    state DRIVE
      en: PRNDMode = 3
    REVERSE -> NEUTRAL [order 1] : [ Neutral || ...
        |   Park || ...
        |   !RunMode]
    NEUTRAL -> REVERSE [order 2] : [ RunMode && ...
        |   Reverse && ...
        |   (Spd <= SpdLoThr) ]
    REVERSE -> DRIVE [order 2] : [ Drive && ...
        |   Spd <= SpdLoThr ]
    DRIVE -> REVERSE [order 2] : [ Reverse && ...
        |   Spd <= SpdLoThr ]
    DRIVE -> NEUTRAL [order 1] : [ Neutral || ...
        |   Park || ...
        |   !RunMode ]
    NEUTRAL -> DRIVE [order 1] : [ RunMode && ...
        |   Drive && ...
        |   (Spd <= SpdLoThr) ]
  (default) -> PARK
  PARK -> REVERSE [order 1] : [ Reverse && ...
      |   AllowShiftFromPark && ...
      |   RunMode ]
  PARK -> NEUTRAL [order 2] : [ Neutral ]
  PARK -> DRIVE [order 3] : [ Drive && ...
      |   AllowShiftFromPark && ...
      |   RunMode ]
  NOT_PARK -> PARK : [ (Park && ...
      |   (Spd <= SpdZeroThr))||ChgMode]
  data: PRNDMode output uint8 size=1; Park input; Reverse input; Neutral input; Drive input; AllowShiftFromPark input; RunMode input; Spd input; SpdZeroThr input; SpdLoThr input; ChgMode input boolean

== stateflow chart VCMGCM1962020b_v2/Fgnd/Control/Modes/Startup & Shutdown/Startup//Shutdown Sequence ==
  state VCM_ON
    en: VCMOn = 1
    state HV_OFF
      en: Step = 0.2
      en: HVSysOff = 1
      ex: HVSysOff = 0
      en: Tmr = 1
      du: Tmr ++
      en, du: ChgCycle = ...
      WakeChgr
    state HV_SHUTDOWN
      state MODULES_OFF
        en: Step = 1.3
        en: ModWake = 0
        en: RunCntr = 0
        en: ChgCntr = 0
      state OPEN_MAIN_CNTRS
        en: Step = 1.2
        en: MainCntr = 0
        en: HVDschg = 1
        ex: HVDschg = 0
      state WAIT2
        en: Step = 1.1
        en: Tmr = 1
        du: Tmr ++
      state WAIT1
        en: Step = 1.0
        en: RampDown = 1
        ex: RampDown = 0
      OPEN_MAIN_CNTRS -> MODULES_OFF : [ HVNoDetect ]
      WAIT2 -> OPEN_MAIN_CNTRS : [ !WaitToDsbl2 || ...
          |   (Tmr >= ...
          |   WaitToDsbl2MxTime) ]
      WAIT1 -> WAIT2 : [ !WaitToDsbl1 ]
    state HV_STARTUP_CHARGE
      state MODULES_ON
        en: Step = 2.0
        en: ModWake = 1
        en: Tmr = 1
        du: Tmr ++
      state CLOSE_CHRG_CNTR
        en:Step=2.05
        en: ChgCntr=1
        en: Tmr = 1
        du: Tmr ++
      state CLOSE_MAIN_CNTRS
        en: Step = 2.1
        en: MainCntr = 1
      state CHARGE
        en: Step = 2.2
        en: Chg = 1
        ex: Chg = 0
        en: Tmr = 1
        du: Tmr ++
      VCM_ON.HV_STARTUP_CHARGE.MODULES_ON -> (junction 262) : [ Tmr >= StartupTimeChg ]
      (junction 262) -> CLOSE_CHRG_CNTR [order 1] : [ HVChgReqd || ...
          |   LVChgReqd ]
          | { MinChgTimeReqd = ...
          |   LVChgReqd;
          |   Tmr = 1 }
      CLOSE_CHRG_CNTR -> VCM_ON.HV_STARTUP_CHARGE.CLOSE_MAIN_CNTRS : [ChrgCntrsFB ==1 && ...
          | Tmr >= SubCntrWait ]
      VCM_ON.HV_STARTUP_CHARGE.CLOSE_MAIN_CNTRS -> CHARGE : [ MainCntrClosed ]
      CHARGE -> VCM_ON.HV_STARTUP_CHARGE.CLOSE_MAIN_CNTRS [order 2] : [ !MainCntrClosed ]
    state HV_STARTUP_RUN
      state MODULES_ON
        en: Step = 3.0
        en: ModWake = 1
        en: Tmr = 1
        du: Tmr ++
      state CLOSE_Run_CNTRs
        en: Step = 3.1
        en: RunCntr = 1
        en: Tmr = 1
        du: Tmr ++
      state CLOSE_MAIN_CNTRS
        en: Step = 3.2
        en: MainCntr = 1
      state RUN
        en: Step = 3.3
        en: Run = 1
        ex: Run = 0
      VCM_ON.HV_STARTUP_RUN.MODULES_ON -> CLOSE_Run_CNTRs : [ Tmr >= StartupTimeRun ]
      CLOSE_Run_CNTRs -> VCM_ON.HV_STARTUP_RUN.CLOSE_MAIN_CNTRS : [ RunCntrFB && ...
          | Tmr >= SubCntrWait]
      VCM_ON.HV_STARTUP_RUN.CLOSE_MAIN_CNTRS -> RUN : [ MainCntrClosed ]
      RUN -> VCM_ON.HV_STARTUP_RUN.CLOSE_MAIN_CNTRS : [ !MainCntrClosed ]
    state DIAGNOSTICS_ENABLE
      en: Step = 0.1
      state OUTPUT_DIAG_ENABLE [parallel]
        settings: executionOrder=2
        state WAIT
        state DELAY
          en: Tmr2 = 1
          du: Tmr2 ++
        state ENABLE
          en: OutptDiagEnbl = 1
        (default) -> WAIT
        WAIT -> VCM_ON.DIAGNOSTICS_ENABLE.OUTPUT_DIAG_ENABLE.DELAY : [ MPRD ]
        VCM_ON.DIAGNOSTICS_ENABLE.OUTPUT_DIAG_ENABLE.DELAY -> VCM_ON.DIAGNOSTICS_ENABLE.OUTPUT_DIAG_ENABLE.ENABLE : [ Tmr2 >= OutptDiagThr ]
      state INPUT_DIAG_ENABLE [parallel]
        settings: executionOrder=1
        state DELAY
          en: Tmr = 1
          du: Tmr ++
        state ENABLE
          en: InptDiagEnbl = 1
        (default) -> VCM_ON.DIAGNOSTICS_ENABLE.INPUT_DIAG_ENABLE.DELAY
        VCM_ON.DIAGNOSTICS_ENABLE.INPUT_DIAG_ENABLE.DELAY -> VCM_ON.DIAGNOSTICS_ENABLE.INPUT_DIAG_ENABLE.ENABLE : [ Tmr >= InptDiagThr ]
      state CAN_DIAG_ENABLE [parallel]
        settings: executionOrder=3
        state DELAY
          en: Tmr3 = 1
          du: Tmr3 ++
        state ENABLE
          en: CANDiagEnbl = 1
        (default) -> VCM_ON.DIAGNOSTICS_ENABLE.CAN_DIAG_ENABLE.DELAY
        VCM_ON.DIAGNOSTICS_ENABLE.CAN_DIAG_ENABLE.DELAY -> VCM_ON.DIAGNOSTICS_ENABLE.CAN_DIAG_ENABLE.ENABLE : [ Tmr3 >= CANDiagThr ]
    HV_OFF -> (junction 301) [order 2] : [ !HVStartupDsbl && ...
        |   !HVDsbl && ...
        |   (!ChgCycle || ...
        |    !WaitReqd || ...
        |   (Tmr >= WaitTime)) ]
    (junction 301) -> (junction 304) [order 2] : { WaitReqd = 0 }
    (junction 301) -> VCM_ON.HV_STARTUP_CHARGE.MODULES_ON [order 1] : [ ChgCycle ]
        | { WaitReqd = 1 }
    (junction 304) -> VCM_ON.HV_STARTUP_RUN.MODULES_ON
    (junction 430) -> HV_OFF
    DIAGNOSTICS_ENABLE -> (junction 430) [order 2] : [ InptDiagEnbl && ...
        |   OutptDiagEnbl && ...
        |   CANDiagEnbl ]
    MODULES_OFF -> HV_OFF
    HV_SHUTDOWN -> HV_OFF : [ !HVDsbl && ...
        |   !FullHVShtdwnReqd ]
    (junction 545) -> MODULES_OFF
    (junction 276) -> (junction 545)
    (junction 262) -> (junction 276) [order 2]
    (junction 315) -> WAIT1
    CHARGE -> (junction 289) [order 1] : [ !HVChgReqd && ...
        |   (!MinChgTimeReqd || ...
        |   (Tmr >= LVChgTime)) ]
        | { FullHVShtdwnReqd = 1 }
    HV_STARTUP_CHARGE -> (junction 282) : [ HVDsbl ]
        | { FullHVShtdwnReqd = 0
        |   WaitReqd = 0 }
    HV_STARTUP_RUN -> (junction 283) : [ HVDsbl ]
        | { FullHVShtdwnReqd = 0 }
    (junction 289) -> (junction 315)
    (junction 282) -> (junction 289)
    (junction 283) -> (junction 282)
  state VCM_OFF
    en: Step = 0.0
    en: VCMOn = 0
    en: InptDiagEnbl = 0
    en: OutptDiagEnbl = 0
    en: CANDiagEnbl = 0
    en: HVSysOff = 1
    en: ChgCycle = 0
    en: ModWake = 0
    en: RunCntr = 0
    en: ChgCntr = 0
    en: MainCntr = 0
    en: Chg = 0
    en: Run = 0
    en: RampDown = 0
    en: HVDschg = 0
    en: WaitReqd = 0
  HV_OFF -> (junction 130) [order 1] : [ Off && ...
      |   Tmr >= ShutdownTime ]
  (junction 130) -> (junction 135)
  DIAGNOSTICS_ENABLE -> (junction 135) [order 1] : [ Off ]
  (junction 135) -> VCM_OFF
  (default) -> VCM_OFF
  VCM_OFF -> DIAGNOSTICS_ENABLE : [ On ]
  data: Step output double size=1; On input; Off input; InptDiagThr input; MPRD input; OutptDiagThr input; CANDiagThr input; WakeChgr input; StartupTimeChg input; StartupTimeRun input; MainCntrClosed input; HVChgReqd input; LVChgReqd input; LVChgTime input; HVStartupDsbl input; Tmr local uint32 size=1; HVDsbl input; WaitToDsbl1 input; WaitToDsbl2 input; WaitToDsbl2MxTime input; HVNoDetect input; VCMOn output boolean size=1; InptDiagEnbl output boolean size=1; OutptDiagEnbl output boolean size=1; CANDiagEnbl output boolean size=1; HVSysOff output boolean size=1; ChgCycle output boolean size=1; ModWake output boolean size=1; MainCntr output boolean size=1; WaitReqd local boolean size=1; Chg output boolean size=1; Run output boolean size=1; RampDown output boolean size=1; HVDschg output boolean size=1; WaitTime input; MinChgTimeReqd local boolean size=1; Tmr2 local uint32 size=1; Tmr3 local uint32 size=1; ShutdownTime input; FullHVShtdwnReqd local boolean size=1; RunCntr output boolean; RunCntrFB input boolean; ChgCntr output boolean; ChrgCntrsFB input; SubCntrWait input

== stateflow chart VCMGCM1962020b_v2/Fgnd/Control/PDU/Main  Contactor Cmd/PreCharge Sequence ==
  state ENABLE
    state Command
      en: CntrCmd = 1
      en: Tmr = 1
      du: Tmr ++
      en: Count ++
    state FAULT
      en: CntrCmd = 0
      en: Tmr = 1
      du: Tmr ++
    state COMPLETE
      en: Complete = 1
    (default) -> Command
    (junction 33) -> Command
    FAULT -> (junction 33) : [ Tmr >= RetryWaitTime && ...
        |   Count < MxAttempts ]
    Command -> COMPLETE [order 2] : [ HVDetect ]
        | { EvalDiag(0) }
    Command -> (junction 29) [order 1] : [ Tmr >= MxTime ]
        | { EvalDiag(1) }
    (junction 29) -> FAULT
  state DISABLE
    en: Complete = 0
    en: CntrCmd = 0
    en: Count = 0
  state EvalDiag(status) [function]
  (default) -> DISABLE
  DISABLE -> ENABLE : [ Enbl ]
  ENABLE -> DISABLE : [ !Enbl ]
  data: status function_input; Complete output boolean size=1; Tmr local uint16 size=1; Enbl input; HVDetect input; MxTime input; RetryWaitTime input; MxAttempts input; Count local uint16 size=1; CntrCmd output boolean

== stateflow chart VCMGCM1962020b_v2/Fgnd/Control/Drive Inverter/Motor Torque Request/Driver Torque Request/Cruise Control/Setpoint/Setpoint ==
  state ON
    state ACTV
      en: Setpt = Spd
      du: Setpt = min(max(Setpt, SetptMn), SetptMx)
      state NORMAL
        en: Actv = 1
        state HOLD_SETPT
          en: State = 2
        state TAP_UP
          en: State = 5
          en: Tmr = 1
          du: Tmr ++
        state TAP_DOWN
          en: State = 3
          en: Tmr = 1
          du: Tmr ++
        state ACCEL
          en: State = 6
          en: Setpt0 = Setpt
          du: Setpt += AccInc
          ex: Setpt = ...
          max(Setpt0, Spd)
        state DECEL
          en: State = 4
          en: Actv = 0
          en: Setpt0 = Setpt
          du: Setpt = ...
          min(Setpt0, Spd)
          ex: Actv = 1
        (default) -> HOLD_SETPT
        HOLD_SETPT -> TAP_DOWN [order 1] : [ hasChangedTo(SetCst,true) ]
        (junction 23) -> HOLD_SETPT
        HOLD_SETPT -> TAP_UP [order 2] : [ hasChangedTo(RsmAcc,true) ]
        TAP_UP -> (junction 23) [order 1] : [ !RsmAcc ]
            | { Setpt = ...
            |   Setpt + TapInc }
        (junction 99) -> (junction 23) [order 2] : { Setpt = ...
            |   Setpt - TapInc }
        TAP_DOWN -> (junction 99) [order 1] : [ !SetCst ]
        (junction 99) -> (junction 23) [order 1] : [ Spd > ...
            |   Setpt + DecDeltaMx ]
            | { Setpt = Spd }
        (junction 26) -> (junction 23)
        TAP_UP -> ACCEL [order 2] : [ Tmr >= TapThr ]
        TAP_DOWN -> DECEL [order 2] : [ Tmr >= TapThr ]
        DECEL -> (junction 26) : [ !SetCst ]
        ACCEL -> (junction 26) : [ !RsmAcc ]
      state STANDBY
        en: State = 7
        en: Actv = 0
      (default) -> NORMAL
      STANDBY -> NORMAL [order 2] : [ SetCst && ...
          |   !Standby ]
          | { Setpt = Spd }
      NORMAL -> STANDBY : [ Standby ]
      STANDBY -> NORMAL [order 1] : [ RsmAcc && ...
          |   !Standby ]
    state INACTV
      en: State = 1
      en: Actv = 0
      en: Setpt = 0
    (default) -> INACTV
    INACTV -> ACTV : [ Enbl && !Standby && ...
        |   SetCst]
    ACTV -> INACTV : [ !Enbl ]
  state OFF
    en: State = 0
    en: Actv = 0
    en: Setpt = 0
  (default) -> OFF
  OFF -> ON : [ On ]
  ON -> OFF : [ !On ]
  data: State output uint8 size=1; Enbl input; Standby input; Spd input; Actv output boolean size=1; Setpt output double size=1; On input; SetCst input; RsmAcc input; TapThr input; DecDeltaMx input; TapInc input; AccInc input; Tmr local uint16 size=1; SetptMx input; SetptMn input; Setpt0 local double size=1

== stateflow chart VCMGCM1962020b_v2/Fgnd/Diagnostics/Diagnostics/HVIL X-Check/EvalDiag/HVIL X-Check ==
  state SUSPECTED
    state TIME
      en: Tmr = 1
      du: Tmr ++
    state FAILED
      en,du: EvalDiag(1)
    (default) -> TIME
    TIME -> FAILED : [ Tmr >= FaultTimeThr ]
  state NOT_SUSPECTED
    en,du: EvalDiag(0)
  state EvalDiag(Status) [function]
  (default) -> (junction 76)
  (junction 76) -> SUSPECTED [order 1] : [ Sus ]
  (junction 76) -> NOT_SUSPECTED [order 2]
  NOT_SUSPECTED -> SUSPECTED : [ Sus ]
  SUSPECTED -> NOT_SUSPECTED : [ !Sus]
  data: Status function_input; Sus input; Tmr local uint16 size=1; FaultTimeThr input
